simulink subsystem "MPC01_nlpsol"  (R2022b)
settings: Solver=VariableStepAuto  StartTime=0.0  StopTime=10.0  RelTol=1e-3
undefined symbols (not defined in the file): param_MPC01, param_traj_data, param_weight_init
settings Model: Creator=emu  LastModifiedBy=emu
settings OptimizationCC: ReuseModelBlockBuffer=on

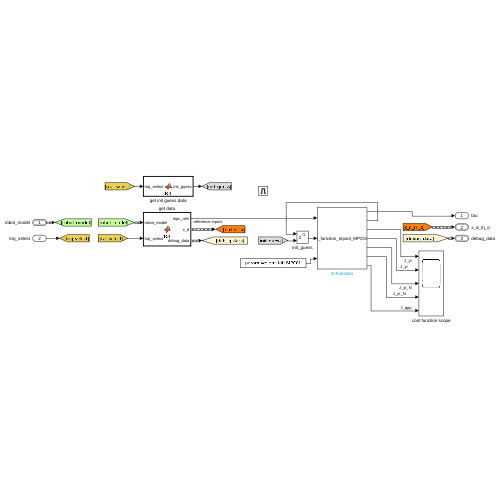
[thumbnail: Simulink's stored preview of the top-level diagram]
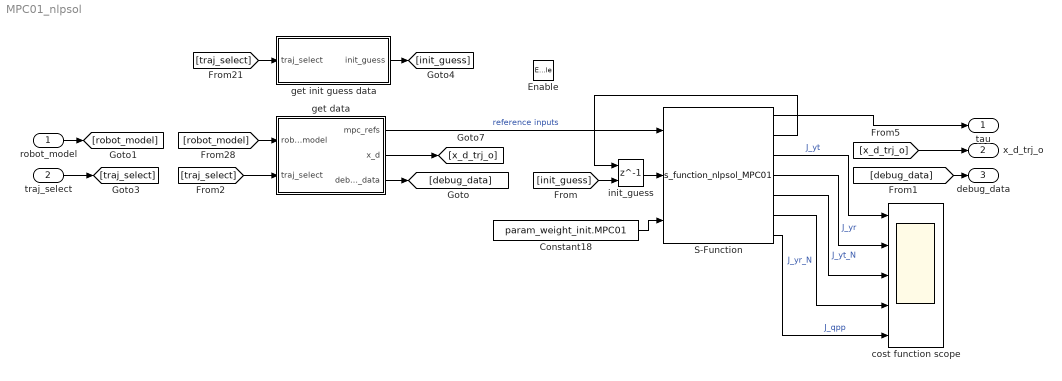
== system MPC01_nlpsol ==
  robot_model : Inport  OutDataTypeStr=Bus: robot_model
  traj_select : Inport  Port=2
  Enable : EnablePort
  Constant18 : Constant  Value=param_weight_init.MPC01  VectorParams1D=off
  S-Function : S-Function  FunctionName=s_function_nlpsol_MPC01  Parameters='s_functions/s_functions_7dof/MPC01.casadi', 'MPC01'  SFunctionModules='MPC01'  SFunctionDeploymentMode=off  EnableBusSupport=off
  cost function scope : Scope  NumInputPorts=5
  get data : MATLAB Function  TreatAsAtomicUnit=on
  get init guess data : MATLAB Function  TreatAsAtomicUnit=on
  init_guess : Delay  DelayLength=1  InitialConditionSource=Input port  InitialCondition=1
      settings: InputPortMap=u0,p4
  tau : Outport
  x_d_trj_o : Outport  Port=2  OutDataTypeStr=Bus: x_d
  debug_data : Outport  Port=3  OutDataTypeStr=Bus: debug_data_bus
  wires:
  robot_model/1 -> [robot_model]
  Constant18/1 -> S-Function/3
  get data/3(debug_data) -> [debug_data]
  get data/1(mpc_refs) -> S-Function/1  "reference inputs"
  [traj_select] -> get init guess data/1(traj_select)
  get init guess data/1(init_guess) -> [init_guess]
  traj_select/1 -> [traj_select]
  [traj_select] -> get data/2(traj_select)
  S-Function/1 -> tau/1
  get data/2(x_d) -> [x_d_trj_o]
  [init_guess] -> init_guess/2
  S-Function/2 -> init_guess/1
  init_guess/1 -> S-Function/2
  S-Function/7 -> cost function scope/5  "J_qpp"
  [x_d_trj_o] -> x_d_trj_o/1
  [robot_model] -> get data/1(robot_model)
  [debug_data] -> debug_data/1
  S-Function/4 -> cost function scope/2  "J_yr"
  S-Function/3 -> cost function scope/1  "J_yt"
  S-Function/6 -> cost function scope/4  "J_yr_N"
  S-Function/5 -> cost function scope/3  "J_yt_N"

== matlab function MPC01_nlpsol/get data ==
  settings: updateMethod=DISCRETE  sampleTime=param_global.Ta
  data: mpc_refs output; robot_model input Bus: robot_model; param_MPC01 parameter; x_d output Bus: x_d; debug_data output Bus: debug_data_bus; param_traj_data parameter; traj_select input
function [mpc_refs, x_d, debug_data] = fcn(robot_model, param_MPC01, param_traj_data, traj_select)
persistent cnt;

if(isempty(cnt))
    cnt = 1;
end

param_MPC = param_MPC01;
N         = param_MPC.N;
N_step    = param_MPC.N_step;

% Parameters
q    = robot_model.q;      % generalized coordinates
q_p  = robot_model.q_p;  % time derivative of generalized coordinates
q_pp = robot_model.q_pp;
H    = robot_model.H;
J    = robot_model.J;
J_p  = robot_model.J_p;

R = H(1:3,1:3);% desired Orientation as rotational matrix
R_d = param_traj_data.R_d(:,:, cnt, traj_select);
q_d = param_traj_data.q_d(:, cnt, traj_select);

%y_q_err = quat_mult(y_q_e, quat_inv(param_traj_data.q_d(1:4, cnt, traj_select)));
q_err = rotation2quaternion(R*R_d');
%y_q_e = rotation2quaternion(R);
q_e = quat_mult(q_d, q_err);

% Current Pose of Endeffector
y = [H(1:3,4); q_e];
y_p = J*q_p;
y_pp = J*q_pp + J_p*q_p;

x_k = [q;q_p];

% Assemble vector of recieved output measurements
p_d    = param_traj_data.p_d(   1:3, cnt : N_step : cnt + (N)*N_step, traj_select);
%p_d_p  = param_traj_data.p_d_p( 1:3, cnt : N_step : cnt + (N)*N_step, traj_select);
%p_d_pp = param_traj_data.p_d_pp(1:3, cnt : N_step : cnt + (N)*N_step, traj_select);

% RPY XYZ angles
%Phi_d    = param_traj_data.Phi_d(      1:3, cnt : N_step : cnt + (N) * N_step, traj_select ); % (Phi_0 ... Phi_N)
%Phi_d_p  = param_traj_data.Phi_d_p(  1:3, cnt : N_step : cnt + (N) * N_step, traj_select ); % (Phi_p_0 ... Phi_p_N)
%Phi_d_pp = param_traj_data.Phi_d_pp(1:3, cnt : N_step : cnt + (N) * N_step, traj_select ); % (Phi_pp_0 ... Phi_pp_N)

q_d       = param_traj_data.q_d(      1:4, cnt : N_step : cnt + (N)*N_step, traj_select);
%omega_d   = param_traj_data.omega_d(  1:3, cnt : N_step : cnt + (N)*N_step, traj_select);
%omega_d_p = param_traj_data.omega_d_p(1:3, cnt : N_step : cnt + (N)*N_step, traj_select);

y_d = [p_d; q_d];            % y_d_1, y_2, ... y_d_N
%y_d_p = [p_d_p; Phi_d_p];    % y_d_p_1, y_2, ... y_d_p_N
%y_d_pp = [p_d_pp; Phi_d_pp]; % y_d_pp_1, y_2, ... y_d_p_N

%% Reference out
mpc_refs = [x_k(:); y_d(:)];

%% TRAJECTORY OUT
x_d.p_d       = param_traj_data.p_d(1:3, cnt, traj_select);    %y0
x_d.p_d_p     = param_traj_data.p_d_p(1:3, cnt, traj_select);  %y0p
x_d.p_d_pp    = param_traj_data.p_d_pp(1:3, cnt, traj_select); %y0pp
x_d.Phi_d     = param_traj_data.Phi_d(:, cnt, traj_select);
x_d.Phi_d_p   = param_traj_data.Phi_d_p(:, cnt, traj_select);
x_d.Phi_d_pp  = param_traj_data.Phi_d_pp(:,cnt, traj_select);
x_d.R_d       = param_traj_data.R_d(:,:, cnt, traj_select);
x_d.q_d       = param_traj_data.q_d(1:4, cnt, traj_select);
x_d.q_d_p     = param_traj_data.q_d_p(1:4, cnt, traj_select);
x_d.q_d_pp    = param_traj_data.q_d_pp(1:4, cnt, traj_select);
x_d.omega_d   = param_traj_data.omega_d(1:3, cnt, traj_select);
x_d.omega_d_p = param_traj_data.omega_d_p(1:3, cnt, traj_select);
x_d.alpha_d    = 0;
x_d.alpha_d_p  = 0;
x_d.alpha_d_pp = 0;
x_d.rot_ax_d   = [0; 0; 0];
x_d.alpha_d_offset = 0;
x_d.q_d_rel = [0; 0; 0; 0];

%% DEBUG
debug_data.p           = y(1:3);
debug_data.p_p         = y_p(1:3);
debug_data.p_pp        = y_pp(1:3);
debug_data.Phi     = rotm2eul_v2(R);
debug_data.Phi_p   = [0; 0; 0]; % ??????
debug_data.Phi_pp  = [0; 0; 0]; % ??????
debug_data.q           = y(4:7);
debug_data.omega       = y_p(4:6);
debug_data.omega_p     = y_pp(4:6);
debug_data.p_err       = y(1:3) - param_traj_data.p_d(:, cnt, traj_select);
debug_data.p_p_err     = y_p(1:3) - param_traj_data.p_d_p(:, cnt, traj_select);
debug_data.p_pp_err    = y_pp(1:3) - param_traj_data.p_d_pp(:, cnt, traj_select);
debug_data.q_err       = q_err;
debug_data.omega_err   = y_p(4:6)  - param_traj_data.omega_d(1:3, cnt, traj_select);
debug_data.omega_p_err = y_pp(4:6) - param_traj_data.omega_d_p(1:3, cnt, traj_select);

cnt = cnt+1;

== matlab function MPC01_nlpsol/get init guess data ==
  data: traj_select input; param_MPC01_init_guess parameter; init_guess output
function init_guess  = fcn(traj_select, param_MPC01_init_guess)

init_guess = param_MPC01_init_guess.init_guess(traj_select,:);
